simulink model "Hybrid_vehicle"  (R2020b)
settings: Solver=FixedStepAuto  StartTime=0.0  StopTime=50  FixedStep=0.001  MaxStep=0.05  RelTol=1e-8
values from neighbouring files (symbols this model uses):
  Bdy_facTireFric_C = 0.018    [Hybrid_vehicle.sldd]
  Bdy_lenRadiusWheel_C = 0.32    [Hybrid_vehicle.sldd]
  Bdy_mEquivalentJ_C = 60.0    [Hybrid_vehicle.sldd]
  Bdy_mVeh_C = 1400.0    [Hybrid_vehicle.sldd]
  Bdy_vsqr2frc_C = 0.429    [Hybrid_vehicle.sldd]
  Drv_facSlopeWLTC_CUR = 0.0 500.0 1000.0 1500.0 2000.0 2500.0 3000.0 3500.0 4000.0 4500.0 5000.0 5500.0 6000.0 6500.0 7000.0 7500.0 8000.0 8500.0 9000.0 9500.0 10000.0 10500.0 11000.0 11500.0 12000.0 12500.0 13000.0 13500.0 14000.0 14500.0 15000.0 15500.0 16000.0 16500.0 17000.0 17500.0 18000.0 18500.0 19000.0 19500.0 20000.0 20500.0 21000.0 21500.0 22000.0 22500.0 23000.0 23500.0 24000.0 0.0 0.01 0.02 0.03 0.04 0.05 0.0    [Hybrid_vehicle.sldd]
  Drv_kmh2gradtqDriver_C = 200.0    [Hybrid_vehicle.sldd]
  Drv_kmh2tqDriver_C = 500.0    [Hybrid_vehicle.sldd]
  Drv_kmhDesWLTC_CUR = 1.0 2.0 3.0 4.0 5.0 6.0 7.0 8.0 9.0 10.0 11.0 12.0 13.0 14.0 15.0 16.0 17.0 18.0 19.0 20.0 21.0 22.0 23.0 24.0 25.0 26.0 27.0 28.0 29.0 30.0 31.0 32.0 33.0 34.0 35.0 36.0 37.0 38.0 39.0 40.0 41.0 42.0 43.0 44.0 45.0 46.0 47.0 48.0 49.0 50.0 51.0 52.0 53.0 54.0 55.0 56.0 57.0 58.0 59.0 60.0 61.0 62.0 63.0 64.0 65.0 66.0 67.0 68.0 69.0 70.0 71.0 72.0 73.0 74.0 75.0 76.0 77.0 78.0 79.0 80.0 81.0 82.0    [Hybrid_vehicle.sldd]
  Edr_pwr_LossMap_AXIS = -150000.0 -100000.0 -60000.0 -35000.0 -23000.0 -7000.0 -2000.0 -1000.0 -200.0 0.0 200.0 1000.0 2000.0 7000.0 23000.0 35000.0 60000.0 100000.0 150000.0    [Hybrid_vehicle.sldd]
  Edr_pwrInverterLosses_MAP = 19500.0 13000.0 6600.0 3500.0 2990.0 1470.0 600.0 450.0 160.0 50.0 160.0 450.0 600.0 1470.0 2530.0 3605.0 6000.0 12000.0 18000.0 15000.0 10000.0 4800.0 2800.0 2300.0 1260.0 600.0 450.0 160.0 50.0 160.0 450.0 600.0 1260.0 1840.0 2555.0 4200.0 9000.0 13500.0 6000.0 4000.0 3000.0 2100.0 1610.0 1050.0 600.0 450.0 160.0 50.0 160.0 450.0 600.0 1050.0 1610.0 2100.0 3000.0 4000.0 6000.0 4500.0 3000.0 2400    [Hybrid_vehicle.sldd]
  Edr_pwrMachineLosses_MAP = 330.0 270.0 210.0 150.0 120.0 90.0 60.0 30.0 10.0 0.0 20.0 40.0 70.0 100.0 130.0 160.0 220.0 280.0 340.0 1797.0 1394.9 1004.3 628.3 452.4 292.8 148.7 51.7 20.3 10.0 19.8 51.4 144.9 283.6 465.1 689.4 1261.5 2017.6 2932.2 2921.3 2122.5 1378.1 724.7 494.3 301.6 158.3 57.8 26.1 18.0 25.9 59.3 156.0 298.6 480.9 668.7 1286.8 2065.9 3033.6 3068.7 2118.7 1325.3 741.4 512.7 329.2 184.3 91.3 45.2 25.0 36.4    [Hybrid_vehicle.sldd]
  Edr_rpm_InvLossMap_AXIS = 0.0 2000.0 5000.0 12000.0    [Hybrid_vehicle.sldd]
  Edr_rpm_MachLossMap_AXIS = 0.0 100.0 200.0 400.0 1000.0 2000.0 4000.0 6000.0 8000.0 10000.0 12000.0    [Hybrid_vehicle.sldd]
  Edr_rpm_MaxMinTq_AXIS = 0.0 100.0 200.0 400.0 1000.0 2000.0 4000.0 5000.0 6000.0 7000.0 8000.0 10000.0 12000.0    [Hybrid_vehicle.sldd]
  Edr_tq_MachLossMap_AXIS = -220.0 -180.0 -140.0 -100.0 -80.0 -60.0 -40.0 -20.0 -10.0 0.0 10.0 20.0 40.0 60.0 80.0 100.0 140.0 180.0 220.0    [Hybrid_vehicle.sldd]
  Edr_tqEffMax_CUR = 220.0 220.0 220.0 220.0 220.0 220.0 220.0 180.0 150.0 125.0 106.0 81.0 65.0    [Hybrid_vehicle.sldd]
  GbxFr_tqClutchMax_C = 500.0    [Hybrid_vehicle.sldd]
  GbxRe_facGbxReRatio_C = 10.0    [Hybrid_vehicle.sldd]
  Ice_derfacLoadDecrease_MAP = -5.0 -200.0 -225.0 -250.0 -275.0 -300.0 -325.0 -350.0 -375.0 -400.0 -10.0 -400.0 -450.0 -500.0 -550.0 -600.0 -650.0 -700.0 -750.0 -800.0 -11.0 -440.0 -495.0 -550.0 -605.0 -660.0 -715.0 -770.0 -825.0 -880.0 -12.0 -480.0 -540.0 -600.0 -660.0 -720.0 -780.0 -840.0 -900.0 -960.0 -13.0 -520.0 -585.0 -650.0 -715.0 -780.0 -845.0 -910.0 -975.0 -1040.0 -14.0 -560.0 -630.0 -700.0 -770.0 -840.0 -910.0 -980.0    [Hybrid_vehicle.sldd]
  Ice_derfacLoadIncrease_MAP = 500.0 30.0 30.0 30.0 30.0 30.0 0.0 0.0 0.0 0.0 500.0 50.0 30.0 30.0 30.0 30.0 30.0 0.0 0.0 0.0 500.0 50.0 15.0 20.0 20.0 20.0 20.0 20.0 0.0 0.0 500.0 50.0 15.0 15.0 18.0 20.0 20.0 20.0 20.0 0.0 500.0 60.0 25.0 20.0 25.0 35.0 40.0 40.0 40.0 0.0 500.0 80.0 30.0 25.0 30.0 40.0 50.0 70.0 70.0 0.0 600.0 90.0 35.0 35.0 45.0 60.0 80.0 100.0 150.0 0.0 800.0 100.0 50.0 40.0 60.0 100.0 150.0 200.0 300.0 0.0    [Hybrid_vehicle.sldd]
  Ice_facEtaCocMax_MAP = 1.0 1.0 0.98 0.955 0.93 1.0 1.0 0.986 0.965 0.94 1.0 1.0 0.995 0.975 0.95 1.0 1.0 1.0 0.985 0.96 1.0 1.0 1.0 0.99 0.97 1.0 1.0 1.0 0.995 0.98 1.0 1.0 1.0 0.998 0.99    [Hybrid_vehicle.sldd]
  Ice_facFuelEnRich_MAP = 1.0 1.0 1.0 1.0 1.0 1.0 1.0 1.0 1.0 1.02 1.0 1.0 1.0 1.0 1.05 1.0 1.0 1.0 1.02 1.08 1.0 1.0 1.0 1.05 1.12 1.0 1.0 1.0 1.08 1.17 1.0 1.0 1.04 1.11 1.25    [Hybrid_vehicle.sldd]
  Ice_Load2TqOptIgnLamOne_MAP = 0.0 35.0 70.0 105.0 140.0 0.0 38.0 76.0 114.0 152.0 0.0 40.0 80.0 120.0 160.0 0.0 40.0 80.0 120.0 160.0 0.0 40.0 80.0 120.0 160.0 0.0 40.0 80.0 120.0 160.0 0.0 40.0 80.0 120.0 160.0    [Hybrid_vehicle.sldd]
  Ice_relLoad_AXIS = 0.0 40.0 80.0 120.0 160.0    [Hybrid_vehicle.sldd]
  Ice_relLoad_LoadDyn_AXIS = 0.0 80.0 90.0 100.0 110.0 120.0 130.0 140.0 150.0 160.0    [Hybrid_vehicle.sldd]
  Ice_relLoad_Max_CUR = 50.0 130.0 137.0 143.0 148.0 153.0 159.0 160.0 160.0 157.0 130.0 90.0    [Hybrid_vehicle.sldd]
  Ice_rpm_AXIS = 0.0 1000.0 2000.0 3000.0 4000.0 5000.0 6000.0    [Hybrid_vehicle.sldd]
  Ice_rpm_LoadDyn_AXIS = 500.0 1000.0 1100.0 1200.0 1300.0 1400.0 1600.0 2400.0 3000.0 4000.0 5000.0 6000.0    [Hybrid_vehicle.sldd]
  Ice_tq_AXIS = 0.0 40.0 80.0 120.0 160.0    [Hybrid_vehicle.sldd]
  Ice_tqLossesIce_MAP = 15.0 13.0 11.0 11.0 11.0 15.0 13.0 11.0 11.0 11.0 16.0 14.0 12.0 12.0 12.0 19.0 17.0 15.0 15.0 15.0 23.0 21.0 19.0 19.0 19.0 29.0 27.0 25.0 25.0 25.0 36.0 34.0 32.0 32.0 32.0    [Hybrid_vehicle.sldd]
  Ice_TqOptIgnLamOne2Load_MAP = 0.0 45.7 91.4 137.14 182.85 0.0 42.1 84.2 126.3 168.4 0.0 40.0 80.0 120.0 160.0 0.0 40.0 80.0 120.0 160.0 0.0 40.0 80.0 120.0 160.0 0.0 40.0 80.0 120.0 160.0 0.0 40.0 80.0 120.0 160.0    [Hybrid_vehicle.sldd]
  Pnt_capBat_C = 54000.0    [Hybrid_vehicle.sldd]
  Pnt_facSocInit_C = 0.6    [Hybrid_vehicle.sldd]
  Pnt_resBatInner_C = 0.2    [Hybrid_vehicle.sldd]
libraries: simulink x2
(part 2 of 2)

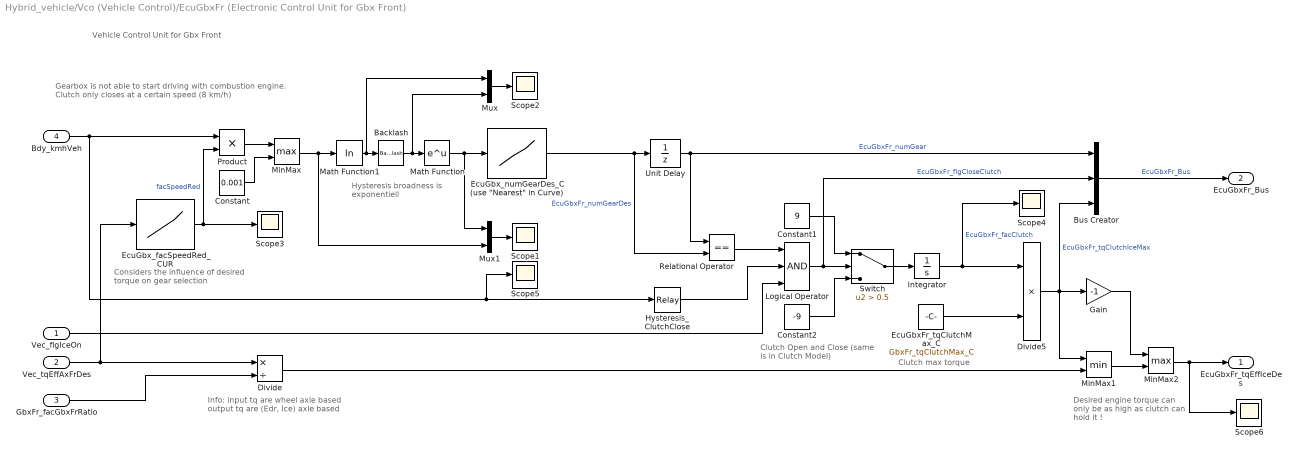
== system Hybrid_vehicle/Vco (Vehicle Control)/EcuGbxFr (Electronic Control Unit for Gbx Front) ==
  note: Gearbox is not able to start driving with combustion engine.
      | Clutch only closes at a certain speed (8 km/h)
  note: Vehicle Control Unit for Gbx Front
  note: Info:
      | input tq are wheel axle based
      | output tq are (Edr, Ice) axle based
  note: Considers the influence of
      | desired torque on gear selection
  note: Hysteresis broadness
      | is exponentiell
  note: Clutch Open and Close
      | (same is in Clutch Model)
  note: Desired engine torque can
      | only be as high as clutch
      | can hold it !
  note: Clutch max torque
  Vec_flgIceOn : Inport
  Vec_tqEffAxFrDes : Inport  Port=2
  GbxFr_facGbxFrRatio : Inport  Port=3
  Bdy_kmhVeh : Inport  Port=4
  Backlash : Backlash  BacklashWidth=0.5  InitialOutput=0.5
  Bus Creator : BusCreator  Inputs=3
  Constant : Constant  Value=0.001
  Constant1 : Constant  Value=9
  Constant2 : Constant  Value=-9
  Divide : Product  Inputs=*/
  Divide5 : Product  Inputs=**
  EcuGbxFr_tqClutchMax_C : Constant  Value=GbxFr_tqClutchMax_C
  EcuGbx_facSpeedRed_CUR : Lookup_n-D  NumberOfTableDimensions=1  BreakpointsForDimension1="[0  50  100 200 300 400 500]"  Table="[1.10  1.03  0.98  0.9  0.85  0.8  0.8 ]"  InternalRulePriority=Speed  RndMeth=Simplest  InputSameDT=on
  "EcuGbx_numGearDes_C (use \"Nearest\" in Curve) " : Lookup_n-D  NumberOfTableDimensions=1  BreakpointsForDimension1="[-0.1  14 25    35     55    80  90  ]"  Table="[1   1         2              3            4          5   5 ]"  InterpMethod=Nearest  InternalRulePriority=Speed  RndMeth=Simplest  InputSameDT=on
  Gain : Gain  Gain=-1
  Hysteresis_ClutchClose : Relay  OnSwitchValue=8  OffSwitchValue=7.5
  Integrator : Integrator  LimitOutput=on  UpperSaturationLimit=1  LowerSaturationLimit=0
  Logical Operator : Logic  Inputs=3  AllPortsSameDT=off  OutDataTypeStr=boolean
  Math Function : Math  SignedPower=on  SaturateOnIntegerOverflow=on
  Math Function1 : Math  Operator=log  SignedPower=on  SaturateOnIntegerOverflow=on
  MinMax : MinMax  Function=max  Inputs=2
  MinMax1 : MinMax  Inputs=2
  MinMax2 : MinMax  Function=max  Inputs=2
  Mux : Mux  Inputs=2
  Mux1 : Mux  Inputs=2
  Product : Product
  Relational Operator : RelationalOperator  Operator===  OutDataTypeStr=boolean  RndMeth=Simplest
  Scope{1..6} (6 alike) : Scope
  Switch : Switch  Criteria=u2 > Threshold  Threshold=0.5
  Unit Delay : UnitDelay  SampleTime=0.2  HasFrameUpgradeWarning=on
  EcuGbxFr_tqEffIceDes : Outport  VectorParamsAs1DForOutWhenUnconnected=off
  EcuGbxFr_Bus : Outport  Port=2  VectorParamsAs1DForOutWhenUnconnected=off
  wires:
  Bus Creator/1 -> EcuGbxFr_Bus/1  "EcuGbxFr_Bus"
  Vec_tqEffAxFrDes/1 -> Divide/1, EcuGbx_facSpeedRed_CUR/1
  Divide/1 -> MinMax1/2
  GbxFr_facGbxFrRatio/1 -> Divide/2
  "EcuGbx_numGearDes_C (use \"Nearest\" in Curve) "/1 -> Relational Operator/2, Unit Delay/1  "EcuGbxFr_numGearDes"
  Backlash/1 -> Mux/2, Math Function/1
  Bdy_kmhVeh/1 -> Hysteresis_ClutchClose/1, Scope5/1, Product/1
  Math Function1/1 -> Mux/1, Backlash/1
  EcuGbx_facSpeedRed_CUR/1 -> Scope3/1, Product/2  "facSpeedRed"
  MinMax/1 -> Math Function1/1, Mux1/2
  Math Function/1 -> Mux1/1, "EcuGbx_numGearDes_C (use \"Nearest\" in Curve) "/1
  Mux/1 -> Scope2/1
  Mux1/1 -> Scope1/1
  Product/1 -> MinMax/1
  Constant/1 -> MinMax/2
  Unit Delay/1 -> Bus Creator/1, Relational Operator/1  "EcuGbxFr_numGear"
  Constant1/1 -> Switch/1
  Switch/1 -> Integrator/1
  Logical Operator/1 -> Bus Creator/2, Switch/2  "EcuGbxFr_flgCloseClutch"
  Constant2/1 -> Switch/3
  Relational Operator/1 -> Logical Operator/1
  Hysteresis_ClutchClose/1 -> Logical Operator/2
  Integrator/1 -> Scope4/1, Divide5/1  "EcuGbxFr_facClutch"
  EcuGbxFr_tqClutchMax_C/1 -> Divide5/2
  Divide5/1 -> Gain/1, MinMax1/1, Bus Creator/3  "EcuGbxFr_tqClutchIceMax"
  MinMax2/1 -> EcuGbxFr_tqEffIceDes/1, Scope6/1
  MinMax1/1 -> MinMax2/2
  Gain/1 -> MinMax2/1
  Vec_flgIceOn/1 -> Logical Operator/3

== system Hybrid_vehicle/Vco (Vehicle Control)/EcuGbxRe (Electronic Control Unit for Gbx Rear) ==
  note: Vehicle Control Unit for Gbx Front
  note: Info:
      | input tq are wheel axle based
      | output tq are (Edr, Ice) axle based
  Vec_tqEffAxReDes : Inport
  GbxRe_facGbxReRatio : Inport  Port=2
  Bus Creator : BusCreator  Inputs=1
  Divide : Product  Inputs=*/
  Ground : Ground
  EcuGbxRe_tqEffEdrDes : Outport  VectorParamsAs1DForOutWhenUnconnected=off
  EcuGbxRe_Bus : Outport  Port=2  VectorParamsAs1DForOutWhenUnconnected=off
  wires:
  Bus Creator/1 -> EcuGbxRe_Bus/1  "EcuGbxRe_Bus"
  Vec_tqEffAxReDes/1 -> Divide/1
  GbxRe_facGbxReRatio/1 -> Divide/2
  Divide/1 -> EcuGbxRe_tqEffEdrDes/1
  Ground/1 -> Bus Creator/1  "test"

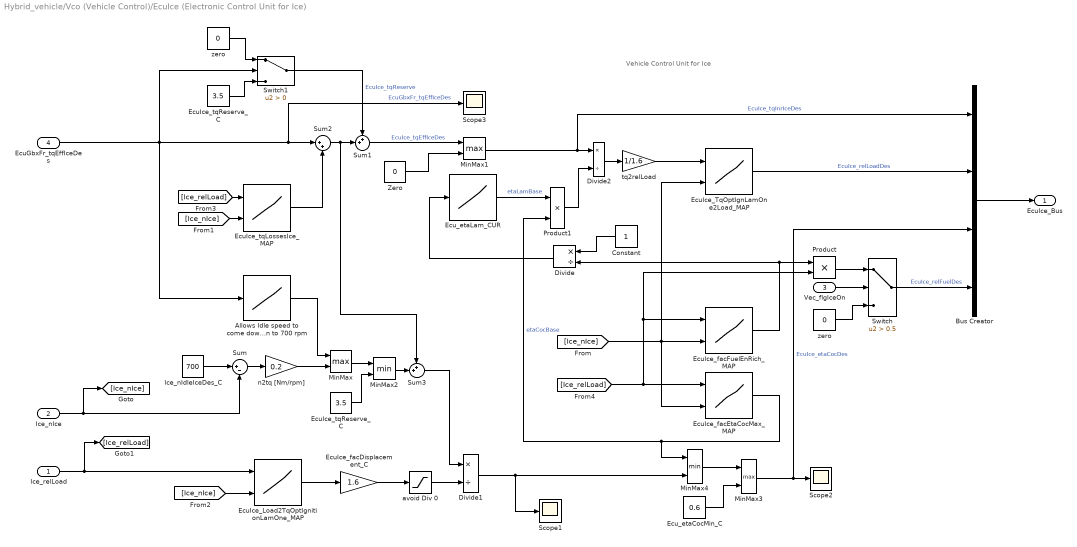
== system Hybrid_vehicle/Vco (Vehicle Control)/EcuIce (Electronic Control Unit for Ice) ==
  note: Vehicle Control Unit for Ice
  Ice_relLoad : Inport
  Ice_nIce : Inport  Port=2
  Vec_flgIceOn : Inport  Port=3
  EcuGbxFr_tqEffIceDes : Inport  Port=4
  " zero " : Constant  Value=0
  Allows Idle speed to come down to 700 rpm : Lookup_n-D  NumberOfTableDimensions=1  BreakpointsForDimension1="[-1 0  1  2]"  Table=[-1 -1 0 0 ]  InternalRulePriority=Speed  RndMeth=Simplest  InputSameDT=on
  Bus Creator : BusCreator  Inputs=4
  Constant : Constant
  Divide : Product  Inputs=*/
  Divide1 : Product  Inputs=*/
  Divide2 : Product  Inputs=*/
  EcuIce_Load2TqOptIgnitionLamOne_MAP : Lookup_n-D  BreakpointsForDimension1=Ice_relLoad_AXIS  BreakpointsForDimension2=Ice_rpm_AXIS  Table=Ice_Load2TqOptIgnLamOne_MAP  ExtrapMethod=Clip  InternalRulePriority=Speed  RndMeth=Simplest  InputSameDT=on
      settings: InputPortMap=u0,u1
  EcuIce_TqOptIgnLamOne2Load_MAP : Lookup_n-D  BreakpointsForDimension1=Ice_tq_AXIS  BreakpointsForDimension2=Ice_rpm_AXIS  Table=Ice_TqOptIgnLamOne2Load_MAP  ExtrapMethod=Clip  InternalRulePriority=Speed  RndMeth=Simplest  InputSameDT=on
      settings: InputPortMap=u0,u1
  EcuIce_facDisplacement_C : Gain  Gain=1.6
  EcuIce_facEtaCocMax_MAP : Lookup_n-D  BreakpointsForDimension1=Ice_relLoad_AXIS  BreakpointsForDimension2=Ice_rpm_AXIS  Table=Ice_facEtaCocMax_MAP  ExtrapMethod=Clip  InternalRulePriority=Speed  RndMeth=Simplest  InputSameDT=on
      settings: InputPortMap=u0,u1
  EcuIce_facFuelEnRich_MAP : Lookup_n-D  BreakpointsForDimension1=Ice_relLoad_AXIS  BreakpointsForDimension2=Ice_rpm_AXIS  Table=Ice_facFuelEnRich_MAP  ExtrapMethod=Clip  InternalRulePriority=Speed  RndMeth=Simplest  InputSameDT=on
      settings: InputPortMap=u0,u1
  EcuIce_tqLossesIce_MAP : Lookup_n-D  BreakpointsForDimension1=Ice_relLoad_AXIS  BreakpointsForDimension2=Ice_rpm_AXIS  Table=Ice_tqLossesIce_MAP  ExtrapMethod=Clip  InternalRulePriority=Speed  RndMeth=Simplest  InputSameDT=on
      settings: InputPortMap=u0,u1
  EcuIce_tqReserve_C : Constant  Value=3.5
  "EcuIce_tqReserve_C " : Constant  Value=3.5
  Ecu_etaCocMin_C : Constant  Value=0.6
  Ecu_etaLam_CUR : Lookup_n-D  NumberOfTableDimensions=1  BreakpointsForDimension1="[0.5    0.6     0.7   0.8   0.85   0.9   1.0   1.1    1.2    1.3    1.4    1.5    1.6    1.7    1.8    1.9    2.0]"  Table="[0       0.5       1     1.1  1.12  1.06   1.0  0.93  0.85   0.78   0.72    0.66    0.625   0.588  0.3  0.2  0]"  ExtrapMethod=Clip  InternalRulePriority=Speed  RndMeth=Simplest  InputSameDT=on
  Ice_nIdleIceDes_C : Constant  Value=700
  MinMax : MinMax  Function=max  Inputs=2
  MinMax1 : MinMax  Function=max  Inputs=2
  MinMax2 : MinMax  Inputs=2
  MinMax3 : MinMax  Function=max  Inputs=2
  MinMax4 : MinMax  Inputs=2
  Product : Product
  Product1 : Product
  Scope1 : Scope
  Scope2 : Scope
  Scope3 : Scope
  Sum : Sum  Inputs=|+-
  Sum1 : Sum  Inputs=++|
  Sum2 : Sum  Inputs=|++
  Sum3 : Sum  Inputs=++|
  Switch : Switch  Criteria=u2 > Threshold  Threshold=0.5
  Switch1 : Switch  Criteria=u2 > Threshold
  "Zero " : Constant  Value=0
  avoid Div 0 : Saturate  UpperLimit=inf  LowerLimit=0.01
  n2tq [Nm/rpm] : Gain  Gain=0.2
  tq2relLoad : Gain  Gain=1/1.6
  "zero " : Constant  Value=0
  EcuIce_Bus : Outport  VectorParamsAs1DForOutWhenUnconnected=off
  wires:
  Bus Creator/1 -> EcuIce_Bus/1
  EcuGbxFr_tqEffIceDes/1 -> Switch1/2, Scope3/1, Sum2/1, Allows Idle speed to come down to 700 rpm/1  "EcuGbxFr_tqEffIceDes"
  Ice_nIdleIceDes_C/1 -> Sum/1
  Sum1/1 -> MinMax1/1  "EcuIce_tqEffIceDes"
  Sum3/1 -> Divide1/1
  Sum/1 -> n2tq [Nm/rpm]/1
  n2tq [Nm/rpm]/1 -> MinMax/2
  Ice_nIce/1 -> [Ice_nIce], Sum/2
  Ice_relLoad/1 -> EcuIce_Load2TqOptIgnitionLamOne_MAP/1, [Ice_relLoad]
  EcuIce_TqOptIgnLamOne2Load_MAP/1 -> Bus Creator/2  "EcuIce_relLoadDes"
  EcuIce_tqLossesIce_MAP/1 -> Sum2/2
  MinMax1/1 -> Bus Creator/1, Divide2/1  "EcuIce_tqInrIceDes"
  "Zero "/1 -> MinMax1/2
  Allows Idle speed to come down to 700 rpm/1 -> MinMax/1
  Vec_flgIceOn/1 -> Switch/2
  EcuIce_facDisplacement_C/1 -> avoid Div 0/1
  EcuIce_Load2TqOptIgnitionLamOne_MAP/1 -> EcuIce_facDisplacement_C/1
  avoid Div 0/1 -> Divide1/2
  "zero "/1 -> Switch1/1
  EcuIce_tqReserve_C/1 -> Switch1/3
  Switch1/1 -> Sum1/1  "EcuIce_tqReserve"
  Sum2/1 -> Sum3/1, Sum1/2
  Divide1/1 -> Scope1/1, MinMax4/2
  MinMax4/1 -> MinMax3/1
  Ecu_etaCocMin_C/1 -> MinMax3/2
  MinMax3/1 -> Scope2/1, Bus Creator/3  "EcuIce_etaCocDes"
  tq2relLoad/1 -> EcuIce_TqOptIgnLamOne2Load_MAP/1
  [Ice_nIce] -> EcuIce_TqOptIgnLamOne2Load_MAP/2, EcuIce_facEtaCocMax_MAP/2, EcuIce_facFuelEnRich_MAP/2
  [Ice_nIce] -> EcuIce_tqLossesIce_MAP/2
  [Ice_nIce] -> EcuIce_Load2TqOptIgnitionLamOne_MAP/2
  [Ice_relLoad] -> EcuIce_tqLossesIce_MAP/1
  MinMax/1 -> MinMax2/1
  MinMax2/1 -> Sum3/2
  "EcuIce_tqReserve_C "/1 -> MinMax2/2
  Switch/1 -> Bus Creator/4  "EcuIce_relFuelDes"
  EcuIce_facEtaCocMax_MAP/1 -> Product1/2, MinMax4/1  "etaCocBase"
  [Ice_relLoad] -> Product/2, EcuIce_facFuelEnRich_MAP/1, EcuIce_facEtaCocMax_MAP/1
  Divide2/1 -> tq2relLoad/1
  Constant/1 -> Divide/1
  Product1/1 -> Divide2/2
  Ecu_etaLam_CUR/1 -> Product1/1  "etaLamBase"
  Divide/1 -> Ecu_etaLam_CUR/1
  EcuIce_facFuelEnRich_MAP/1 -> Product/1, Divide/2
  Product/1 -> Switch/1
  " zero "/1 -> Switch/3

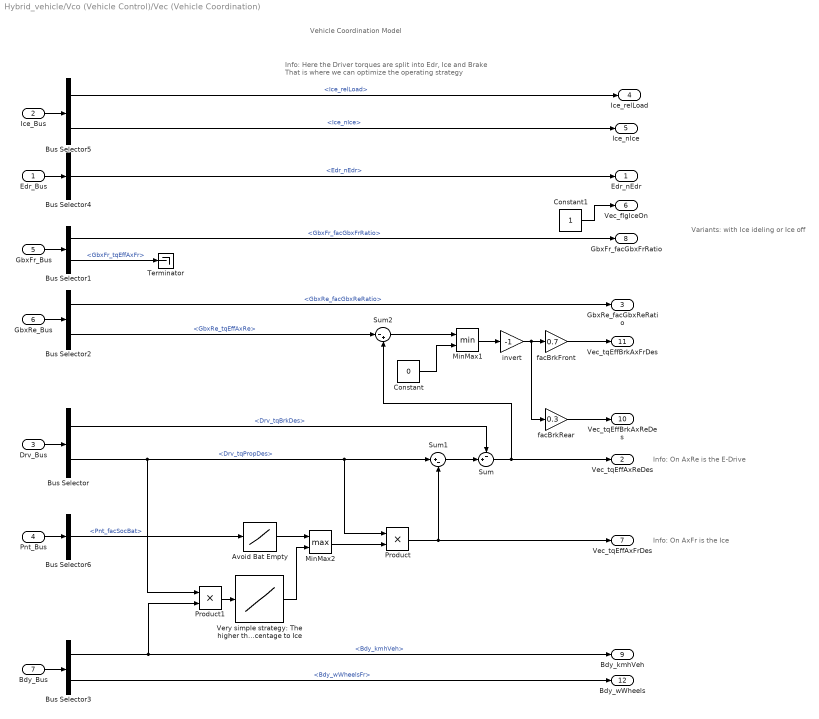
== system Hybrid_vehicle/Vco (Vehicle Control)/Vec (Vehicle Coordination) ==
  note: Vehicle Coordination Model
  note: Info: Here the Driver torques are split into Edr, Ice and Brake
      | That is where we can optimize the operating strategy
  note: Info: On AxRe is the E-Drive
  note: Info: On AxFr is the Ice
  note: Variants: with Ice ideling or Ice off
  Edr_Bus : Inport
  Ice_Bus : Inport  Port=2
  Drv_Bus : Inport  Port=3
  Pnt_Bus : Inport  Port=4
  GbxFr_Bus : Inport  Port=5
  GbxRe_Bus : Inport  Port=6
  Bdy_Bus : Inport  Port=7
  Avoid Bat Empty : Lookup_n-D  NumberOfTableDimensions=1  BreakpointsForDimension1="[0 0.1 0.2  1]"  Table="[1.1 0.8  0 0]"  InternalRulePriority=Speed  RndMeth=Simplest  InputSameDT=on
  Bus Selector : BusSelector  OutputSignals=Drv_tqBrkDes,Drv_tqPropDes
  Bus Selector1 : BusSelector  OutputSignals=GbxFr_facGbxFrRatio,GbxFr_tqEffAxFr
  Bus Selector2 : BusSelector  OutputSignals=GbxRe_facGbxReRatio,GbxRe_tqEffAxRe
  Bus Selector3 : BusSelector  OutputSignals=Bdy_kmhVeh,Bdy_wWheelsFr
  Bus Selector4 : BusSelector  OutputSignals=Edr_nEdr
  Bus Selector5 : BusSelector  OutputSignals=Ice_relLoad,Ice_nIce
  Bus Selector6 : BusSelector  OutputSignals=Pnt_facSocBat
  Constant : Constant  Value=0
  Constant1 : Constant
  MinMax1 : MinMax  Inputs=2  ZeroCross=off
  MinMax2 : MinMax  Function=max  Inputs=2  ZeroCross=off
  Product : Product
  Product1 : Product
  Sum : Sum  Inputs=-+|
  Sum1 : Sum  Inputs=|+-
  Sum2 : Sum  Inputs=|-+
  Terminator : Terminator
  "Very simple strategy: The higher the power, the more percentage to Ice" : Lookup_n-D  NumberOfTableDimensions=1  BreakpointsForDimension1="[0 2000  8000  15000  50000 200000]"  Table="[0 0  0.5 0.7  1 1]"  InternalRulePriority=Speed  RndMeth=Simplest  InputSameDT=on
  facBrkFront : Gain  Gain=0.7
  facBrkRear : Gain  Gain=0.3
  invert : Gain  Gain=-1
  Edr_nEdr : Outport  VectorParamsAs1DForOutWhenUnconnected=off
  Vec_tqEffAxReDes : Outport  Port=2  VectorParamsAs1DForOutWhenUnconnected=off
  GbxRe_facGbxReRatio : Outport  Port=3  VectorParamsAs1DForOutWhenUnconnected=off
  Ice_relLoad : Outport  Port=4  VectorParamsAs1DForOutWhenUnconnected=off
  Ice_nIce : Outport  Port=5  VectorParamsAs1DForOutWhenUnconnected=off
  Vec_flgIceOn : Outport  Port=6  VectorParamsAs1DForOutWhenUnconnected=off
  Vec_tqEffAxFrDes : Outport  Port=7  VectorParamsAs1DForOutWhenUnconnected=off
  GbxFr_facGbxFrRatio : Outport  Port=8  VectorParamsAs1DForOutWhenUnconnected=off
  Bdy_kmhVeh : Outport  Port=9  VectorParamsAs1DForOutWhenUnconnected=off
  Vec_tqEffBrkAxReDes : Outport  Port=10  VectorParamsAs1DForOutWhenUnconnected=off
  Vec_tqEffBrkAxFrDes : Outport  Port=11  VectorParamsAs1DForOutWhenUnconnected=off
  Bdy_wWheels : Outport  Port=12  VectorParamsAs1DForOutWhenUnconnected=off
  wires:
  Drv_Bus/1 -> Bus Selector/1
  Bus Selector/2 -> Sum1/1, Product/1, Product1/1  "<Drv_tqPropDes>"
  Bus Selector/1 -> Sum/1  "<Drv_tqBrkDes>"
  Sum/1 -> Vec_tqEffAxReDes/1, Sum2/2
  GbxFr_Bus/1 -> Bus Selector1/1
  Bus Selector1/1 -> GbxFr_facGbxFrRatio/1  "<GbxFr_facGbxFrRatio>"
  GbxRe_Bus/1 -> Bus Selector2/1
  Bus Selector2/1 -> GbxRe_facGbxReRatio/1  "<GbxRe_facGbxReRatio>"
  Bdy_Bus/1 -> Bus Selector3/1
  Bus Selector3/1 -> Bdy_kmhVeh/1, Product1/2  "<Bdy_kmhVeh>"
  Bus Selector3/2 -> Bdy_wWheels/1  "<Bdy_wWheelsFr>"
  Product/1 -> Vec_tqEffAxFrDes/1, Sum1/2
  Edr_Bus/1 -> Bus Selector4/1
  Bus Selector4/1 -> Edr_nEdr/1  "<Edr_nEdr>"
  Sum2/1 -> MinMax1/1
  MinMax1/1 -> invert/1
  Ice_Bus/1 -> Bus Selector5/1
  facBrkFront/1 -> Vec_tqEffBrkAxFrDes/1
  invert/1 -> facBrkRear/1, facBrkFront/1
  facBrkRear/1 -> Vec_tqEffBrkAxReDes/1
  Constant/1 -> MinMax1/2
  Sum1/1 -> Sum/2
  Bus Selector2/2 -> Sum2/1  "<GbxRe_tqEffAxRe>"
  Bus Selector5/1 -> Ice_relLoad/1  "<Ice_relLoad>"
  Bus Selector5/2 -> Ice_nIce/1  "<Ice_nIce>"
  Product1/1 -> "Very simple strategy: The higher the power, the more percentage to Ice"/1
  Constant1/1 -> Vec_flgIceOn/1
  Pnt_Bus/1 -> Bus Selector6/1
  Bus Selector6/1 -> Avoid Bat Empty/1  "<Pnt_facSocBat>"
  MinMax2/1 -> Product/2
  "Very simple strategy: The higher the power, the more percentage to Ice"/1 -> MinMax2/2
  Avoid Bat Empty/1 -> MinMax2/1
  Bus Selector1/2 -> Terminator/1  "<GbxFr_tqEffAxFr>"
